simulink model "clutchLockUp"  (R2020b)
settings: Solver=VariableStepAuto  StartTime=0.0  StopTime=10.0  RelTol=1e-3
values from neighbouring files (symbols this model uses):
  be = 2    [constant.m]
  bv = 1    [constant.m]
  le = 1    [constant.m]
  lv = 5    [constant.m]
  muk = 1    [constant.m]
  R = 1    [constant.m]
settings Model: Creator=shraddha  LastModifiedBy=shraddha

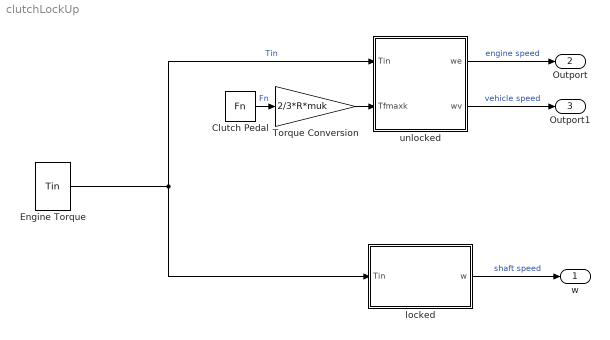
== system clutchLockUp ==
  Clutch Pedal : FromWorkspace  VariableName=Fn  ZeroCross=off
  Engine Torque : FromWorkspace  VariableName=Tin  ZeroCross=off
  Torque Conversion : Gain  Gain=2/3*R*muk  SaturateOnIntegerOverflow=on  OutDataTypeStr=Inherit: Same as input  ParamDataTypeStr=Inherit: Same as input
  locked : Subsystem
  unlocked : Subsystem
  w : Outport
  Outport : Outport  Port=2
  Outport1 : Outport  Port=3
  wires:
  locked/1(w) -> w/1  "shaft speed"
  Torque Conversion/1 -> unlocked/2(Tfmaxk)
  unlocked/1(we) -> Outport/1  "engine speed"
  unlocked/2(wv) -> Outport1/1  "vehicle speed"
  Clutch Pedal/1 -> Torque Conversion/1  "Fn"
  Engine Torque/1 -> locked/1(Tin), unlocked/1(Tin)  "Tin"

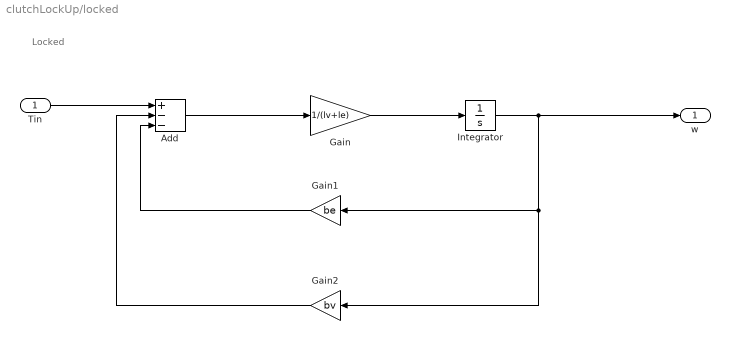
== system clutchLockUp/locked ==
  note: Locked
  Tin : Inport
  Add : Sum  Inputs=+--
  Gain : Gain  Gain=1/(lv+le)
  Gain1 : Gain  Gain=be
  Gain2 : Gain  Gain=bv
  Integrator : Integrator
  w : Outport
  wires:
  Integrator/1 -> w/1, Gain1/1, Gain2/1
  Gain2/1 -> Add/2
  Add/1 -> Gain/1
  Tin/1 -> Add/1
  Gain1/1 -> Add/3
  Gain/1 -> Integrator/1

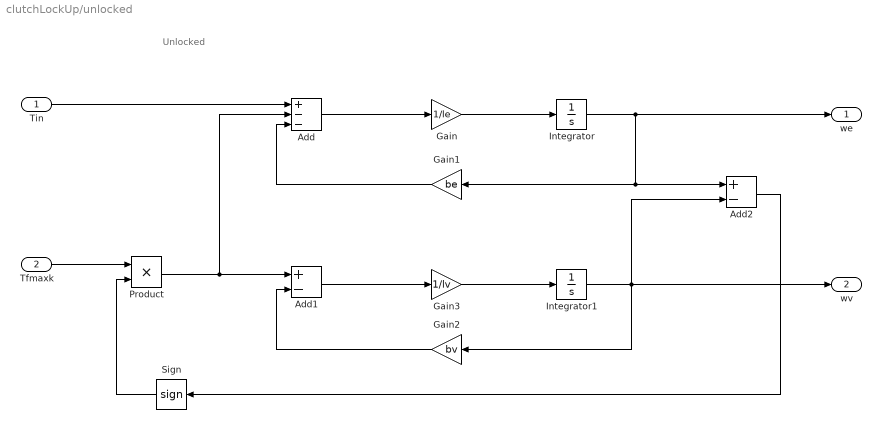
== system clutchLockUp/unlocked ==
  note: Unlocked
  Tin : Inport
  Tfmaxk : Inport  Port=2
  Add : Sum  Inputs=+--
  Add1 : Sum  Inputs=+-
  Add2 : Sum  Inputs=+-
  Gain : Gain  Gain=1/le
  Gain1 : Gain  Gain=be
  Gain2 : Gain  Gain=bv
  Gain3 : Gain  Gain=1/lv
  Integrator : Integrator
  Integrator1 : Integrator
  Product : Product
  Sign : Signum  ZeroCross=off
  we : Outport
  wv : Outport  Port=2
  wires:
  Gain3/1 -> Integrator1/1
  Integrator1/1 -> wv/1, Add2/2, Gain2/1
  Gain/1 -> Integrator/1
  Gain1/1 -> Add/3
  Product/1 -> Add1/1, Add/2
  Gain2/1 -> Add1/2
  Add2/1 -> Sign/1
  Integrator/1 -> we/1, Gain1/1, Add2/1
  Add/1 -> Gain/1
  Sign/1 -> Product/2
  Add1/1 -> Gain3/1
  Tin/1 -> Add/1
  Tfmaxk/1 -> Product/1
